simulink library "wtd_library_ver1"  (R2014b)
settings: Solver=ode45  StartTime=0.0  StopTime=10.0  RelTol=1e-3
undefined symbols (not defined in the file or in its folder): clearaugYMatrix, complexPower, dwo, faultaugYMatrix, genTranReactance, invclearaugYMatrix, invfaultaugYMatrix, invsystemaugYMatrix, j, nodeVoltage, noGridNodes, pffault_set_global, s3cc, tho
undefined symbols (not defined in the file): baseSystemPower, internalGenVoltage, pitchAngleVec, systemFrequency, turbSpeedVec, windturbKaParam, windturbKbParam, WTD_Y12, WTD_Y12_2
libraries: simulink x18
(part 2 of 3)

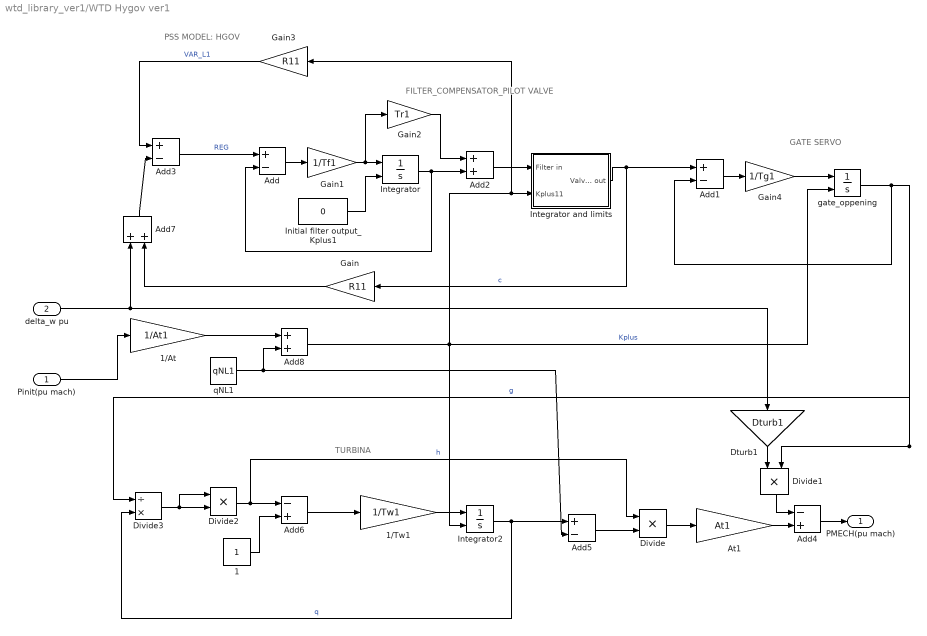
== system wtd_library_ver1/WTD Hygov ver1 ==
  note: GATE SERVO
  note: FILTER_COMPENSATOR_PILOT VALVE
  note: TURBINA
  note: PSS MODEL: HGOV
  Pinit(pu mach) : Inport
  delta_w pu : Inport  Port=2
  1 : Constant
  1/At : Gain  Gain=1/At1
  1/Tw1 : Gain  Gain=1/Tw1
  Add{,1,3,5} (4 alike) : Sum  Inputs=+-
  Add2 : Sum
  Add4 : Sum  Inputs=-+
  Add6 : Sum  Inputs=-+
  Add7 : Sum
  Add8 : Sum
  At1 : Gain  Gain=At1
  Divide : Product  Inputs=**
  Divide1 : Product  Inputs=**
  Divide2 : Product  Inputs=**
  Divide3 : Product  Inputs=/*
  Dturb1 : Gain  Gain=Dturb1
  Gain : Gain  Gain=R11
  Gain1 : Gain  Gain=1/Tf1
  Gain2 : Gain  Gain=Tr1
  Gain3 : Gain  Gain=R11
  Gain4 : Gain  Gain=1/Tg1
  Initial filter output_Kplus1 : Constant  Value=0
  Integrator : Integrator  InitialConditionSource=external  UpperSaturationLimit=VELM1  LowerSaturationLimit=-VELM1
  Integrator and limits : Subsystem
  Integrator2 : Integrator  InitialConditionSource=external
  gate_oppening : Integrator  InitialConditionSource=external
  qNL1 : Constant  Value=qNL1
  PMECH(pu mach) : Outport
  wires:
  Gain3/1 -> Add3/1  "VAR_L1"
  Add8/1 -> Gain3/1, Integrator and limits/2(Kplus11), gate_oppening/2, Integrator2/2  "Kplus"
  1/At/1 -> Add8/1
  Pinit(pu mach)/1 -> 1/At/1
  Gain2/1 -> Add2/1
  Add2/1 -> Integrator and limits/1(Filter in)
  Add/1 -> Gain1/1
  Gain1/1 -> Gain2/1, Integrator/1
  Initial filter output_Kplus1/1 -> Integrator/2
  Integrator/1 -> Add2/2, Add/2
  At1/1 -> Add4/2
  Add4/1 -> PMECH(pu mach)/1
  Divide/1 -> At1/1
  Divide1/1 -> Add4/1
  Add5/1 -> Divide/2
  1/Tw1/1 -> Integrator2/1
  qNL1/1 -> Add8/2, Add5/2
  Integrator2/1 -> Add5/1, Divide3/2  "q"
  Add6/1 -> 1/Tw1/1
  1/1 -> Add6/2
  Divide2/1 -> Add6/1, Divide/1  "h"
  Divide3/1 -> Divide2/2, Divide2/1
  Gain4/1 -> gate_oppening/1
  Add1/1 -> Gain4/1
  Integrator and limits/1(Valve out) -> Add1/1, Gain/1  "c"
  gate_oppening/1 -> Add1/2, Divide3/1, Divide1/2  "g"
  Add3/1 -> Add/1  "REG"
  Add7/1 -> Add3/2
  delta_w pu/1 -> Add7/1, Dturb1/1
  Gain/1 -> Add7/2
  Dturb1/1 -> Divide1/1

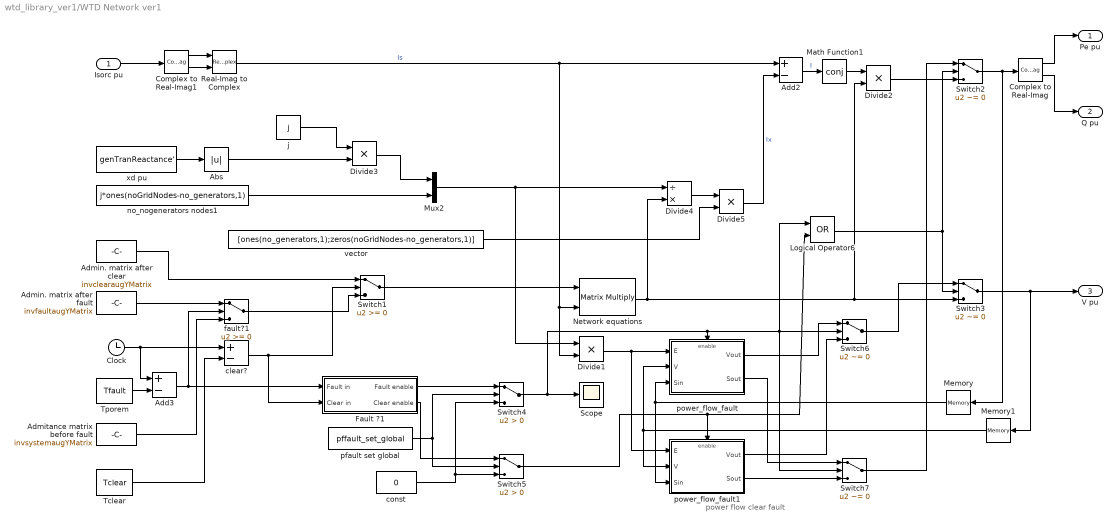
== system wtd_library_ver1/WTD Network ver1 ==
  note: power flow clear fault
  Isorc pu : Inport  OutDataTypeStr=double
  Abs : Abs
  Add2 : Sum  Inputs=+-
  Add3 : Sum  Inputs=+-
  Admin. matrix after fault : Constant  Value=invfaultaugYMatrix
  Admin. matrix after clear : Constant  Value=invclearaugYMatrix
  Admitance matrix before fault : Constant  Value=invsystemaugYMatrix
  Clock : Clock
  Complex to Real-Imag : ComplexToRealImag
  Complex to Real-Imag1 : ComplexToRealImag
  Divide{1..3,5} (4 alike) : Product  Inputs=**
  Divide4 : Product  Inputs=/*
  Fault ?1 : Subsystem
  Logical Operator6 : Logic  Operator=OR  AllPortsSameDT=off  OutDataTypeStr=boolean
  Math Function1 : Math  Operator=conj  SaturateOnIntegerOverflow=on
  Memory : Memory  X0=complexPower
  Memory1 : Memory  X0=nodeVoltage
  Mux2 : Mux  Inputs=2
  Network equations : Product  Inputs=**  Multiplication=Matrix(*)
  Real-Imag to Complex : RealImagToComplex
  Scope : Scope
      settings: MaxDataPoints=50000
  Switch1 : Switch
  Switch{2..3,6..7} (4 alike) : Switch  Criteria=u2 ~= 0
  Switch4 : Switch  Criteria=u2 > Threshold
  Switch5 : Switch  Criteria=u2 > Threshold
  Tclear : Constant  Value=Tclear
  Tporem : Constant  Value=Tfault
  clear? : Sum  Inputs=+-
  const : Constant  Value=0
  fault?1 : Switch
  j : Constant  Value=j
  no_nogenerators nodes1 : Constant  Value=j*ones(noGridNodes-no_generators,1)
  pfault set global : Constant  Value=pffault_set_global
  power_flow_fault : Subsystem
  power_flow_fault1 : Subsystem
  vector : Constant  Value=[ones(no_generators,1);zeros(noGridNodes-no_generators,1)]  VectorParams1D=off
  xd pu : Constant  Value=genTranReactance'
  Pe pu : Outport
  Q pu : Outport  Port=2
  V pu : Outport  Port=3
  wires:
  Divide1/1 -> power_flow_fault/1(E), power_flow_fault1/1(E)
  Divide3/1 -> Mux2/1
  no_nogenerators nodes1/1 -> Mux2/2
  Complex to Real-Imag/2 -> Q pu/1
  Complex to Real-Imag/1 -> Pe pu/1
  Math Function1/1 -> Divide2/1
  Add2/1 -> Math Function1/1  "I"
  Divide5/1 -> Add2/2  "Ix"
  vector/1 -> Divide5/2
  Divide4/1 -> Divide5/1
  Switch1/1 -> Network equations/1
  fault?1/1 -> Switch1/3
  clear?/1 -> Fault ?1/2(Clear in), Switch1/2
  Admin. matrix after clear/1 -> Switch1/1
  Tclear/1 -> clear?/2
  Add3/1 -> fault?1/2, Fault ?1/1(Fault in)
  Tporem/1 -> Add3/2
  Clock/1 -> Add3/1, clear?/1
  Admitance matrix before fault/1 -> fault?1/3
  Admin. matrix after fault/1 -> fault?1/1
  j/1 -> Divide3/1
  Abs/1 -> Divide3/2
  Mux2/1 -> Divide1/1, Divide4/1
  Network equations/1 -> Divide4/2, Divide2/2, Switch3/3
  xd pu/1 -> Abs/1
  Isorc pu/1 -> Complex to Real-Imag1/1
  Complex to Real-Imag1/1 -> Real-Imag to Complex/1
  Complex to Real-Imag1/2 -> Real-Imag to Complex/2
  Real-Imag to Complex/1 -> Add2/1, Network equations/2, Divide1/2  "Is"
  Divide2/1 -> Switch2/3
  Switch2/1 -> Complex to Real-Imag/1, Memory/1
  Switch3/1 -> V pu/1, Memory1/1
  const/1 -> Switch4/3, Switch5/3
  pfault set global/1 -> Switch4/2, Switch5/2
  Switch4/1 -> power_flow_fault/Enable, Logical Operator6/1, Switch6/2, Switch7/2, Scope/1
  Memory/1 -> power_flow_fault/3(Sin), power_flow_fault1/3(Sin)
  Memory1/1 -> power_flow_fault/2(V), power_flow_fault1/2(V)
  Switch5/1 -> power_flow_fault1/Enable, Logical Operator6/2
  Logical Operator6/1 -> Switch2/2, Switch3/2
  power_flow_fault/1(Vout) -> Switch6/1
  power_flow_fault1/1(Vout) -> Switch6/3
  power_flow_fault/2(Sout) -> Switch7/1
  power_flow_fault1/2(Sout) -> Switch7/3
  Switch6/1 -> Switch3/1
  Switch7/1 -> Switch2/1
  Fault ?1/1(Fault enable) -> Switch4/1
  Fault ?1/2(Clear enable) -> Switch5/1

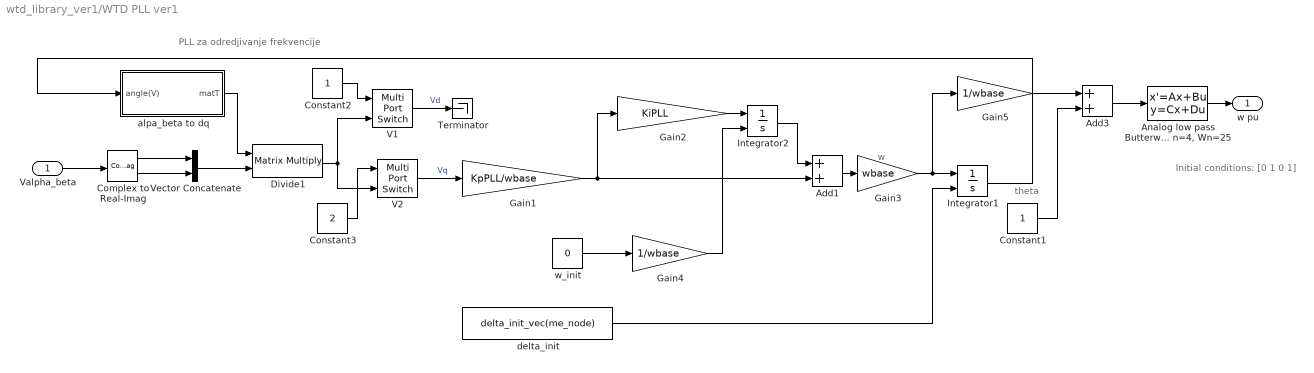
== system wtd_library_ver1/WTD PLL ver1 ==
  note: PLL za odredjivanje frekvencije
  note: theta
  note: w
  note: Initial conditions:
      | [0 1 0 1]
  Valpha_beta : Inport
  Add1 : Sum
  Add3 : Sum
  "Analog low pass Butterworth filter, n=4, Wn=25" : StateSpace  A=[-46.194,-25,0,0;25,0,0,0;0,25,-19.134,-25;0,0,25,0]  B=[25;0;0;0]  C=[0,0,0,1]  D=0  X0=[0 1 0 1]
  Complex to Real-Imag : ComplexToRealImag
  Constant1 : Constant
  Constant2 : Constant
  Constant3 : Constant  Value=2
  Divide1 : Product  Inputs=**  Multiplication=Matrix(*)
  Gain1 : Gain  Gain=KpPLL/wbase
  Gain2 : Gain  Gain=KiPLL
  Gain3 : Gain  Gain=wbase
  Gain4 : Gain  Gain=1/wbase
  Gain5 : Gain  Gain=1/wbase
  Integrator1 : Integrator  InitialConditionSource=external
  Integrator2 : Integrator  InitialConditionSource=external
  Terminator : Terminator
  V1 : MultiPortSwitch  Inputs=1
  V2 : MultiPortSwitch  Inputs=1
  Vector Concatenate : Concatenate
  alpa_beta to dq : Subsystem
  delta_init : Constant  Value=delta_init_vec(me_node)
  w_init : Constant  Value=0
  w pu : Outport
  wires:
  "Analog low pass Butterworth filter, n=4, Wn=25"/1 -> w pu/1
  Add3/1 -> "Analog low pass Butterworth filter, n=4, Wn=25"/1
  Valpha_beta/1 -> Complex to Real-Imag/1
  alpa_beta to dq/1(matT) -> Divide1/1
  Vector Concatenate/1 -> Divide1/2
  Complex to Real-Imag/1 -> Vector Concatenate/1
  Complex to Real-Imag/2 -> Vector Concatenate/2
  Gain1/1 -> Gain2/1, Add1/2
  Integrator1/1 -> alpa_beta to dq/1(angle(V))
  Constant2/1 -> V1/1
  Constant3/1 -> V2/1
  V1/1 -> Terminator/1  "Vd"
  Add1/1 -> Gain3/1
  Integrator2/1 -> Add1/1
  Gain2/1 -> Integrator2/1
  V2/1 -> Gain1/1  "Vq"
  Gain3/1 -> Integrator1/1, Gain5/1
  delta_init/1 -> Integrator1/2
  Gain4/1 -> Integrator2/2
  Gain5/1 -> Add3/1
  Constant1/1 -> Add3/2
  Divide1/1 -> V1/2, V2/2
  w_init/1 -> Gain4/1

== system wtd_library_ver1/WTD Rotor ver1 ==
  note: This subsystem models the mechanical part of the synchronous machine (Kundur)
  "deltaPe pu mach " : Inport  PortDimensions=1
  deltaPm pu mach : Inport  Port=2  PortDimensions=1
  initial_angle(elrad) : Inport  Port=3  PortDimensions=1
  delta_w_init pu : Inport  Port=4  PortDimensions=1
  Constant : Constant
  F1 : Gain  Gain=D  SaturateOnIntegerOverflow=on  OutDataTypeStr=Inherit: Same as input  ParamDataTypeStr=Inherit: Same as input
  H : Constant  Value=H
  Integrator : Integrator  InitialConditionSource=external  InitialCondition=dwo
  Integrator2 : Integrator  InitialConditionSource=external  InitialCondition=tho
  Product1 : Product  Inputs=*/  SaturateOnIntegerOverflow=on  InputSameDT=on  OutDataTypeStr=Inherit: Same as first input
  Product2 : Product  Inputs=*/  SaturateOnIntegerOverflow=on  InputSameDT=on  OutDataTypeStr=Inherit: Same as first input
  Sum1 : Sum  Inputs=+-  SaturateOnIntegerOverflow=on  InputSameDT=on  OutDataTypeStr=Inherit: Same as first input
  Sum2 : Sum  Inputs=+-  SaturateOnIntegerOverflow=on  InputSameDT=on  OutDataTypeStr=Inherit: Same as first input
  Sum3 : Sum  SaturateOnIntegerOverflow=on  InputSameDT=on  OutDataTypeStr=Inherit: Same as first input
  gain : Gain  Gain=2  SaturateOnIntegerOverflow=on  OutDataTypeStr=Inherit: Same as input  ParamDataTypeStr=Inherit: Same as input
  wbase : Gain  Gain=wbase  SaturateOnIntegerOverflow=on  OutDataTypeStr=Inherit: Same as input  ParamDataTypeStr=Inherit: Same as input
  angle(elrad) : Outport  InitialOutput=0
  "delta_w pu " : Outport  Port=2  InitialOutput=0
  wires:
  "deltaPe pu mach "/1 -> Sum2/2  "Pe"
  Product1/1 -> Integrator/1
  Integrator/1 -> wbase/1, F1/1, "delta_w pu "/1, Sum3/2  "dw"
  wbase/1 -> Integrator2/1  "delta_w"
  Integrator2/1 -> angle(elrad)/1  "delta (rad)"
  initial_angle(elrad)/1 -> Integrator2/2
  delta_w_init pu/1 -> Integrator/2
  H/1 -> gain/1
  gain/1 -> Product1/2
  Sum1/1 -> Product1/1
  F1/1 -> Sum1/2
  Sum2/1 -> Product2/1
  Product2/1 -> Sum1/1
  Constant/1 -> Sum3/1
  Sum3/1 -> Product2/2
  deltaPm pu mach/1 -> Sum2/1

== system wtd_library_ver1/WTD Tgov1 ver1 ==
  note: MODEL PSS: TGOV1
  Pinit(pu mach) : Inport
  delta_w pu : Inport  Port=2
  Add : Sum  Inputs=+-
  Add1 : Sum  Inputs=+-
  Add2 : Sum  Inputs=++-
  Add3 : Sum  Inputs=+-
  Gain : Gain  Gain=1/R2
  Gain1 : Gain  Gain=1/T12
  Gain2 : Gain  Gain=1/T32
  Gain3 : Gain  Gain=T22
  Gain4 : Gain  Gain=Dt2
  Gain5 : Gain  Gain=R2
  Integrator : Integrator  InitialConditionSource=external  LimitOutput=on  UpperSaturationLimit=Vmax2  LowerSaturationLimit=Vmin2
  Integrator1 : Integrator  InitialConditionSource=external
  PMECH(pu mach) : Outport
  wires:
  Pinit(pu mach)/1 -> Gain5/1, Integrator/2, Integrator1/2
  Gain5/1 -> Add3/1
  Add3/1 -> Gain/1
  delta_w pu/1 -> Add3/2, Gain4/1
  Gain4/1 -> Add2/3
  Add2/1 -> PMECH(pu mach)/1
  Gain3/1 -> Add2/1
  Integrator1/1 -> Add2/2, Add1/2
  Gain2/1 -> Gain3/1, Integrator1/1
  Add1/1 -> Gain2/1
  Integrator/1 -> Add1/1, Add/2
  Gain1/1 -> Integrator/1
  Add/1 -> Gain1/1
  Gain/1 -> Add/1

== system wtd_library_ver1/WTD Thermo ver1 ==
  note: STEAM 2
  Pe pu : Inport
  Add4 : Sum  Inputs=+-
  Add5 : Sum  Inputs=+-
  Gain1 : Gain  Gain=1/Sbasem2
  Gain2 : Gain  Gain=Sbasesys/Sbasem2
  Gain3 : Gain  Gain=Sbasem2/Sbasesys
  Pm_init : Constant  Value=Pm_init_vec(co_node)
  Rotor/Load1 : Subsystem
  TGOV1 : Subsystem
  delta_init (elrad) : Constant  Value=delta_init_vec(co_node)
  delta_w2 : Constant  Value=0
  Pm pu : Outport
  angle(elrad) : Outport  Port=2
  delta_w pu : Outport  Port=3
  wires:
  Pm_init/1 -> Gain1/1
  TGOV1/1(PMECH) -> Gain3/1, Add4/1
  Add5/1 -> Rotor/Load1/1("deltaPe(pu) ")
  Add4/1 -> Rotor/Load1/2(deltaPm(pu))
  Rotor/Load1/2(delta_w(pu)) -> TGOV1/2(deltaw), delta_w pu/1
  delta_w2/1 -> Rotor/Load1/4(deltawro)
  Gain2/1 -> Add5/1
  Pe pu/1 -> Gain2/1
  Gain3/1 -> Pm pu/1
  Rotor/Load1/1(delta(elrad)) -> angle(elrad)/1
  delta_init (elrad)/1 -> Rotor/Load1/3(angle(E)(elrad))
  Gain1/1 -> Add4/2, Add5/2, TGOV1/1(Pinit (pu mach))

== system wtd_library_ver1/WTD Vec_ sig_sel ver1 ==
  in : Inport
  V7 : MultiPortSwitch  Inputs=1
  signal node : Constant  Value=node
  out : Outport
  wires:
  in/1 -> V7/2
  V7/1 -> out/1
  signal node/1 -> V7/1

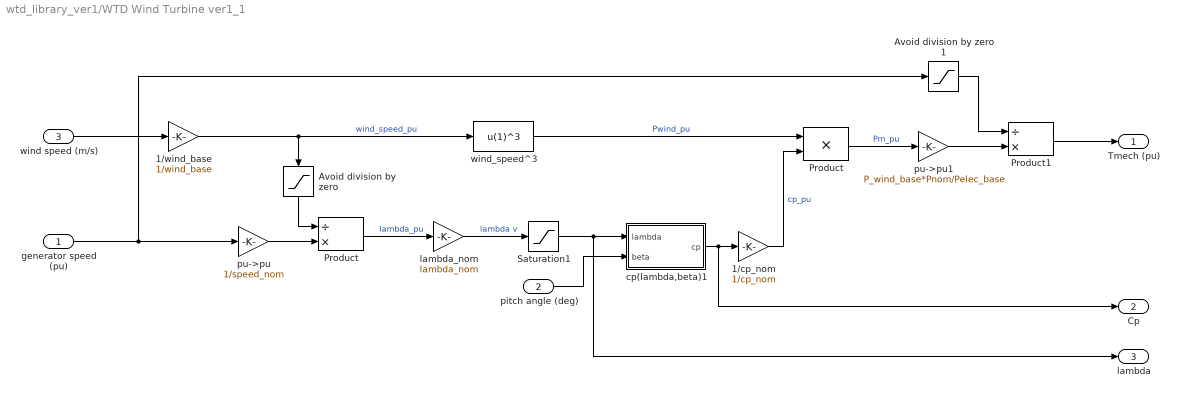
== system wtd_library_ver1/WTD Wind Turbine ver1_1 ==
  generator speed (pu) : Inport
  pitch angle (deg) : Inport  Port=2
  wind speed (m/s) : Inport  Port=3
  1/cp_nom : Gain  Gain=1/cp_nom  SaturateOnIntegerOverflow=on  OutDataTypeStr=Inherit: Same as input  ParamDataTypeStr=Inherit: Same as input
  1/wind_base : Gain  Gain=1/wind_base  SaturateOnIntegerOverflow=on  OutDataTypeStr=Inherit: Same as input  ParamDataTypeStr=Inherit: Same as input
  "Avoid division by zero " : Saturate  UpperLimit=1e6  LowerLimit=1e-6
  Avoid division by zero 1 : Saturate  UpperLimit=1e6  LowerLimit=1e-6
  Product : Product  Inputs=/*  SaturateOnIntegerOverflow=on  OutDataTypeStr=Inherit: Same as first input
  "Product " : Product  SaturateOnIntegerOverflow=on  OutDataTypeStr=Inherit: Same as first input
  Product1 : Product  Inputs=/*  SaturateOnIntegerOverflow=on  OutDataTypeStr=Inherit: Same as first input
  Saturation1 : Saturate  UpperLimit=inf  LowerLimit=1e-6
  cp(lambda,beta)1 : Subsystem
  lambda_nom : Gain  Gain=lambda_nom  SaturateOnIntegerOverflow=on  OutDataTypeStr=Inherit: Same as input  ParamDataTypeStr=Inherit: Same as input
  "pu->pu " : Gain  Gain=1/speed_nom  SaturateOnIntegerOverflow=on  OutDataTypeStr=Inherit: Same as input  ParamDataTypeStr=Inherit: Same as input
  pu->pu1 : Gain  Gain=P_wind_base*Pnom/Pelec_base  SaturateOnIntegerOverflow=on  OutDataTypeStr=Inherit: Same as input  ParamDataTypeStr=Inherit: Same as input
  wind_speed^3 : Fcn  Expr=u(1)^3
  Tmech (pu) : Outport
  Cp : Outport  Port=2
  lambda : Outport  Port=3
  wires:
  wind speed (m/s)/1 -> 1/wind_base/1
  "pu->pu "/1 -> Product/2
  "Avoid division by zero "/1 -> Product/1
  1/wind_base/1 -> "Avoid division by zero "/1, wind_speed^3/1  "wind_speed_pu"
  Product/1 -> lambda_nom/1  "lambda_pu"
  Saturation1/1 -> cp(lambda,beta)1/1(lambda), lambda/1
  1/cp_nom/1 -> "Product "/2  "cp_pu"
  lambda_nom/1 -> Saturation1/1  "lambda v"
  generator speed (pu)/1 -> "pu->pu "/1, Avoid division by zero 1/1
  wind_speed^3/1 -> "Product "/1  "Pwind_pu"
  cp(lambda,beta)1/1(cp) -> Cp/1, 1/cp_nom/1
  pitch angle (deg)/1 -> cp(lambda,beta)1/2(beta)
  Avoid division by zero 1/1 -> Product1/1
  Product1/1 -> Tmech (pu)/1
  pu->pu1/1 -> Product1/2
  "Product "/1 -> pu->pu1/1  "Pm_pu"

== system wtd_library_ver1/WTD zero_gen ver1 ==
  Complex to Real-Imag : ComplexToRealImag
  Constant : Constant  Value=0
  Real-Imag to Complex : RealImagToComplex
  Isorc : Outport
  wires:
  Real-Imag to Complex/1 -> Isorc/1
  Complex to Real-Imag/2 -> Real-Imag to Complex/2
  Complex to Real-Imag/1 -> Real-Imag to Complex/1
  Constant/1 -> Complex to Real-Imag/1

== system wtd_library_ver1/WTD DFIG_ver1/Calculation of Power to network  ==
  absVterm : Inport
  Vterm : Inport  Port=2
  Isorc : Inport  Port=3
  Xsec : Inport  Port=4
  Add1 : Sum  Inputs=+-
  Complex to Real-Imag1 : ComplexToRealImag  Output=Real
  Complex to Real-Imag2 : ComplexToRealImag  Output=Imag
  Divide : Product  Inputs=**
  Divide1 : Product  Inputs=*/
  Divide4 : Product  Inputs=**
  Gain1 : Gain  Gain=-1
  Math Function : Math  Operator=conj  SaturateOnIntegerOverflow=on
  Math Function1 : Math  Operator=square  SaturateOnIntegerOverflow=on
  j : Constant  Value=j
  Pgen=Pelec : Outport
  Qgen : Outport  Port=2
  Sgen : Outport  Port=3
  wires:
  Gain1/1 -> Divide1/2
  Divide4/1 -> Gain1/1
  j/1 -> Divide4/2
  Math Function1/1 -> Divide1/1
  Divide1/1 -> Add1/2
  Divide/1 -> Complex to Real-Imag1/1, Add1/1  "Selec"
  Add1/1 -> Complex to Real-Imag2/1, Sgen/1  "Sgen (after Xsec)"
  Math Function/1 -> Divide/2
  absVterm/1 -> Math Function1/1
  Vterm/1 -> Divide/1
  Isorc/1 -> Math Function/1
  Xsec/1 -> Divide4/1
  Complex to Real-Imag1/1 -> Pgen=Pelec/1  "Pelec"
  Complex to Real-Imag2/1 -> Qgen/1

== system wtd_library_ver1/WTD DFIG_ver1/Converter control model ==
  note: Measurements
  Vrfq : Inport
  Vreg : Inport  Port=2
  Qord_sep_mod : Inport  Port=3
  PFAref : Inport  Port=4
  Pelec : Inport  Port=5
  Qgen : Inport  Port=6
  Vterm : Inport  Port=7
  Pord : Inport  Port=8
  Qinput_droop : Inport  Port=9
  Qref : Inport  Port=10
  Aux_Test_Sig : Inport  Port=11
  Electrical Control : Subsystem
  Reactive Power Control : Subsystem
  Eqcmd : Outport
  Ipcmd : Outport  Port=2
  wires:
  Electrical Control/2(Ipcmd) -> Ipcmd/1
  Electrical Control/1(Eqcmd) -> Eqcmd/1
  Aux_Test_Sig/1 -> Electrical Control/5(Aux_Test_Sig)
  Pord/1 -> Electrical Control/4(Pord)
  Vterm/1 -> Electrical Control/3(Vterm)
  Qgen/1 -> Electrical Control/2(Qgen)
  Reactive Power Control/1(Qcmd) -> Electrical Control/1(Qcmd)
  Qinput_droop/1 -> Reactive Power Control/6(Qinput_droop)
  Qref/1 -> Reactive Power Control/7(Qref)
  Pelec/1 -> Reactive Power Control/5(Pelec)
  PFAref/1 -> Reactive Power Control/4(PFAref)
  Qord_sep_mod/1 -> Reactive Power Control/3(Qord_sep_mod)
  Vreg/1 -> Reactive Power Control/2(Vreg)
  Vrfq/1 -> Reactive Power Control/1(Vrfq)

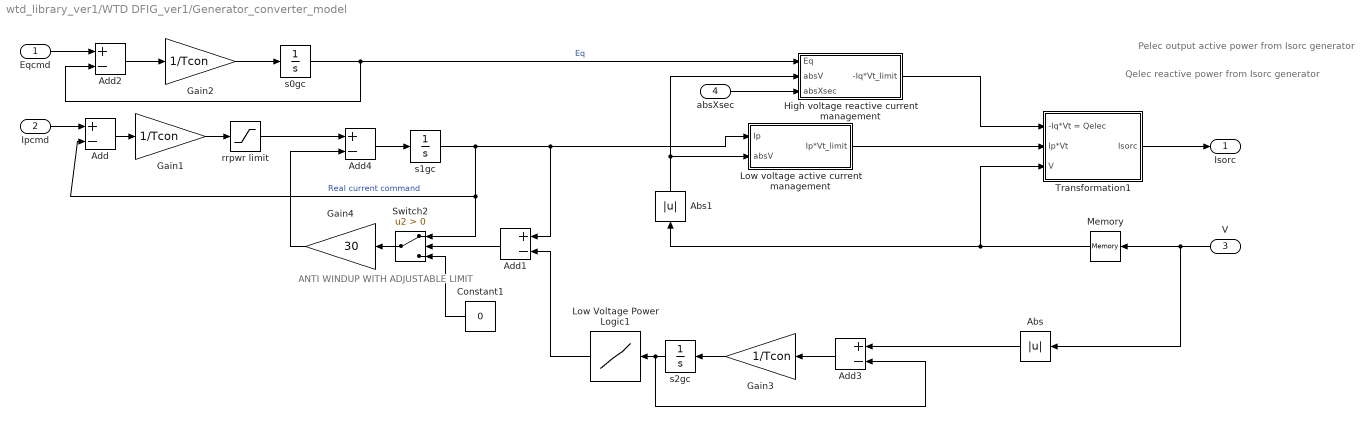
== system wtd_library_ver1/WTD DFIG_ver1/Generator_converter_model ==
  note: Pelec output active power from Isorc generator
  note: Qelec reactive power from Isorc generator
  note: ANTI WINDUP WITH ADJUSTABLE
      | LIMIT
  Eqcmd : Inport
  Ipcmd : Inport  Port=2
  V : Inport  Port=3
  absXsec : Inport  Port=4
  " Transformation1" : Subsystem
  Abs : Abs
  Abs1 : Abs
  Add{,1..4} (5 alike) : Sum  Inputs=+-
  Constant1 : Constant  Value=0
  Gain1 : Gain  Gain=1/Tcon
  Gain2 : Gain  Gain=1/Tcon
  Gain3 : Gain  Gain=1/Tcon
  Gain4 : Gain  Gain=30
  High voltage reactive current management : Subsystem
  Low Voltage Power Logic1 : Lookup  InputValues=[0,zerox,brkpt,brkpt+eps,brkpt+2*eps]  Table=[0 0 1.22 2 2]
  Low voltage active current management : Subsystem
  Memory : Memory  X0=nodeVoltage(co_node)
  Switch2 : Switch  Criteria=u2 > Threshold
  rrpwr limit : Saturate  UpperLimit=rrpwr  LowerLimit=-inf
  s0gc : Integrator  InitialCondition=s0gc
  s1gc : Integrator  InitialCondition=s1gc
  s2gc : Integrator  InitialCondition=s2gc
  Isorc : Outport
  wires:
  Abs/1 -> Add3/1
  " Transformation1"/1(Isorc) -> Isorc/1
  absXsec/1 -> High voltage reactive current management/3(absXsec)
  V/1 -> Abs/1, Memory/1
  Add3/1 -> Gain3/1
  s2gc/1 -> Add3/2, Low Voltage Power Logic1/1
  Gain3/1 -> s2gc/1
  s0gc/1 -> Add2/2, High voltage reactive current management/1(Eq)  "Eq"
  Gain2/1 -> s0gc/1
  Add2/1 -> Gain2/1
  Eqcmd/1 -> Add2/1
  Ipcmd/1 -> Add/1
  Add/1 -> Gain1/1
  Gain1/1 -> rrpwr limit/1
  High voltage reactive current management/1(-Iq*Vt_limit) -> " Transformation1"/1(-Iq*Vt = Qelec)
  Low voltage active current management/1(Ip*Vt_limit) -> " Transformation1"/2(Ip*Vt)
  Abs1/1 -> Low voltage active current management/2(absV), High voltage reactive current management/2(absV)
  s1gc/1 -> Add/2, Switch2/1, Low voltage active current management/1(Ip), Add1/1  "Real current command"
  Memory/1 -> " Transformation1"/3(V), Abs1/1
  rrpwr limit/1 -> Add4/1
  Add4/1 -> s1gc/1
  Switch2/1 -> Gain4/1
  Constant1/1 -> Switch2/3
  Gain4/1 -> Add4/2
  Low Voltage Power Logic1/1 -> Add1/2
  Add1/1 -> Switch2/2

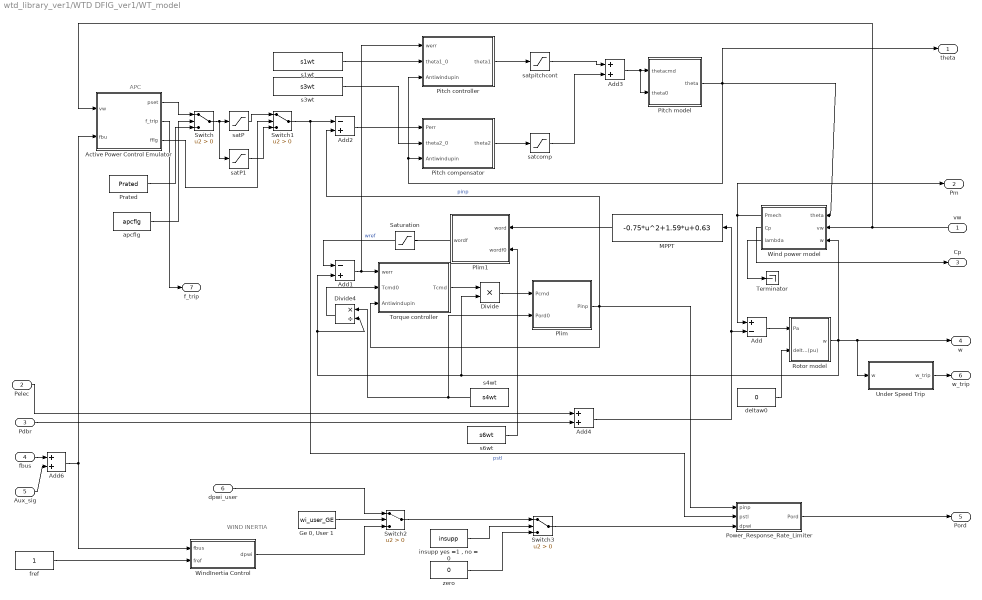
== system wtd_library_ver1/WTD DFIG_ver1/WT_model ==
  note: WIND INERTIA
  note: APC
  vw : Inport
  Pelec : Inport  Port=2
  Pdbr : Inport  Port=3
  fbus : Inport  Port=4
  Aux_sig : Inport  Port=5
  dpwi_user : Inport  Port=6
  Active Power Control Emulator : Subsystem
  Add : Sum  Inputs=+-
  Add1 : Sum  Inputs=-+
  Add2 : Sum  Inputs=-+
  Add3 : Sum
  Add4 : Sum
  Add6 : Sum
  Divide : Product  Inputs=**
  Divide4 : Product  Inputs=*/
  "Ge 0, User 1" : Constant  Value=wi_user_GE
  MPPT : Fcn  Expr=-0.75*u^2+1.59*u+0.63
  Pitch compensator : Subsystem
  Pitch controller : Subsystem
  Pitch model : Subsystem
  Plim : Subsystem
  Plim1 : Subsystem
  Power_Response_Rate_Limiter : Subsystem
  Prated : Constant  Value=Prated
  Rotor model : Subsystem
  Saturation : Saturate  UpperLimit=wrefgr  LowerLimit=0.63
  Switch{,1..3} (4 alike) : Switch  Criteria=u2 > Threshold
  Terminator : Terminator
  Torque controller : Subsystem
  Under Speed Trip : Subsystem
  Wind power model : Subsystem
  WindInertia Control : Subsystem
  apcflg : Constant  Value=apcflg
  deltaw0 : Constant  Value=0
  fref : Constant
  "insupp yes =1 , no = 0" : Constant  Value=insupp
  s1wt : Constant  Value=s1wt
  s3wt : Constant  Value=s3wt
  s4wt : Constant  Value=s4wt
  s6wt : Constant  Value=s6wt
  satP : Saturate  UpperLimit=+inf  LowerLimit=Pmin
  satP1 : Saturate  UpperLimit=Pmax  LowerLimit=Pmin
  satcomp : Saturate  UpperLimit=upltpitchcomp  LowerLimit=lowltpitchcomp
  satpitchcont : Saturate  UpperLimit=upltpitchcont  LowerLimit=lowltpitchcont
  zero : Constant  Value=0
  theta : Outport
  Pm : Outport  Port=2
  Cp : Outport  Port=3
  w : Outport  Port=4
  Pord : Outport  Port=5
  w_trip : Outport  Port=6
  f_trip : Outport  Port=7
  wires:
  Switch3/1 -> Power_Response_Rate_Limiter/3(dpwi)
  zero/1 -> Switch3/3
  Switch2/1 -> Switch3/1
  "insupp yes =1 , no = 0"/1 -> Switch3/2
  deltaw0/1 -> Rotor model/2(deltaw0(pu))
  Power_Response_Rate_Limiter/1(Pord) -> Pord/1
  fref/1 -> WindInertia Control/2(fref)
  WindInertia Control/1(dpwi) -> Switch2/3
  dpwi_user/1 -> Switch2/1
  satP1/1 -> Switch1/3
  satP/1 -> Switch1/1
  Switch1/1 -> Power_Response_Rate_Limiter/2(pstl), Add2/1  "pstl"
  Active Power Control Emulator/3(fflg) -> Switch1/2
  Active Power Control Emulator/2(f_trip) -> f_trip/1
  Under Speed Trip/1(w_trip) -> w_trip/1
  Aux_sig/1 -> Add6/2
  Pdbr/1 -> Add4/2
  Pelec/1 -> Add4/1
  Wind power model/2(Cp) -> Cp/1
  apcflg/1 -> Switch/2
  Prated/1 -> Switch/3
  Active Power Control Emulator/1(pset) -> Switch/1
  Switch/1 -> satP1/1, satP/1
  Add6/1 -> WindInertia Control/1(fbus), Active Power Control Emulator/2(fbu)
  fbus/1 -> Add6/1
  Wind power model/3(lambda) -> Terminator/1
  Add4/1 -> Add/2, MPPT/1
  satcomp/1 -> Add3/2
  satpitchcont/1 -> Add3/1
  Plim1/1(wordf) -> Saturation/1
  MPPT/1 -> Plim1/1(word)
  vw/1 -> Wind power model/2(vw), Active Power Control Emulator/1(vw)
  s1wt/1 -> Pitch controller/2(theta1_0)
  s3wt/1 -> Pitch compensator/2(theta2_0)
  Divide4/1 -> Torque controller/2(Tcmd0)
  s6wt/1 -> Plim1/2(wordf0)
  s4wt/1 -> Plim/2(Pord0), Divide4/1
  Plim/1(Pinp) -> Power_Response_Rate_Limiter/1(pinp), Torque controller/3(Antiwindupin), Add2/2  "pinp"
  Wind power model/1(Pmech) -> Add/1, Pm/1
  Pitch model/1(theta) -> theta/1, Pitch compensator/3(Antiwindupin), Pitch controller/3(Antiwindupin), Wind power model/1(theta)
  Add3/1 -> Pitch model/2(theta0), Pitch model/1(thetacmd)
  Pitch compensator/1(theta2) -> satcomp/1
  Pitch controller/1(theta1) -> satpitchcont/1
  Add2/1 -> Pitch compensator/1(Perr)
  Saturation/1 -> Add1/1  "wref"
  Add1/1 -> Pitch controller/1(werr), Torque controller/1(werr)
  Torque controller/1(Tcmd) -> Divide/1
  Rotor model/1(w) -> Under Speed Trip/1(w), w/1, Divide4/2, Add1/2, Divide/2, Wind power model/3(w)
  Divide/1 -> Plim/1(Pcmd)
  Add/1 -> Rotor model/1(Pa)
  "Ge 0, User 1"/1 -> Switch2/2

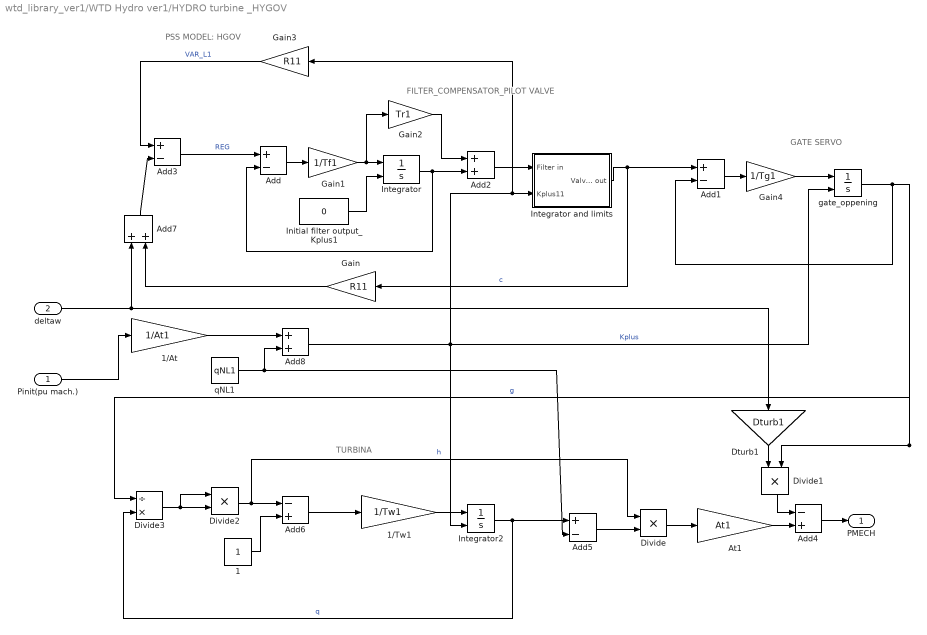
== system wtd_library_ver1/WTD Hydro ver1/HYDRO turbine _HYGOV ==
  note: GATE SERVO
  note: FILTER_COMPENSATOR_PILOT VALVE
  note: TURBINA
  note: PSS MODEL: HGOV
  Pinit(pu mach.) : Inport
  deltaw : Inport  Port=2
  1 : Constant
  1/At : Gain  Gain=1/At1
  1/Tw1 : Gain  Gain=1/Tw1
  Add{,1,3,5} (4 alike) : Sum  Inputs=+-
  Add2 : Sum
  Add4 : Sum  Inputs=-+
  Add6 : Sum  Inputs=-+
  Add7 : Sum
  Add8 : Sum
  At1 : Gain  Gain=At1
  Divide : Product  Inputs=**
  Divide1 : Product  Inputs=**
  Divide2 : Product  Inputs=**
  Divide3 : Product  Inputs=/*
  Dturb1 : Gain  Gain=Dturb1
  Gain : Gain  Gain=R11
  Gain1 : Gain  Gain=1/Tf1
  Gain2 : Gain  Gain=Tr1
  Gain3 : Gain  Gain=R11
  Gain4 : Gain  Gain=1/Tg1
  Initial filter output_Kplus1 : Constant  Value=0
  Integrator : Integrator  InitialConditionSource=external  UpperSaturationLimit=VELM1  LowerSaturationLimit=-VELM1
  Integrator and limits : Subsystem
  Integrator2 : Integrator  InitialConditionSource=external
  gate_oppening : Integrator  InitialConditionSource=external
  qNL1 : Constant  Value=qNL1
  PMECH : Outport
  wires:
  Gain3/1 -> Add3/1  "VAR_L1"
  Add8/1 -> Gain3/1, Integrator and limits/2(Kplus11), gate_oppening/2, Integrator2/2  "Kplus"
  1/At/1 -> Add8/1
  Pinit(pu mach.)/1 -> 1/At/1
  Gain2/1 -> Add2/1
  Add2/1 -> Integrator and limits/1(Filter in)
  Add/1 -> Gain1/1
  Gain1/1 -> Gain2/1, Integrator/1
  Initial filter output_Kplus1/1 -> Integrator/2
  Integrator/1 -> Add2/2, Add/2
  At1/1 -> Add4/2
  Add4/1 -> PMECH/1
  Divide/1 -> At1/1
  Divide1/1 -> Add4/1
  Add5/1 -> Divide/2
  1/Tw1/1 -> Integrator2/1
  qNL1/1 -> Add8/2, Add5/2
  Integrator2/1 -> Add5/1, Divide3/2  "q"
  Add6/1 -> 1/Tw1/1
  1/1 -> Add6/2
  Divide2/1 -> Add6/1, Divide/1  "h"
  Divide3/1 -> Divide2/2, Divide2/1
  Gain4/1 -> gate_oppening/1
  Add1/1 -> Gain4/1
  Integrator and limits/1(Valve out) -> Add1/1, Gain/1  "c"
  gate_oppening/1 -> Add1/2, Divide3/1, Divide1/2  "g"
  Add3/1 -> Add/1  "REG"
  Add7/1 -> Add3/2
  deltaw/1 -> Add7/1, Dturb1/1
  Gain/1 -> Add7/2
  Dturb1/1 -> Divide1/1

== system wtd_library_ver1/WTD Hydro ver1/Rotor//Load2 ==
  note: This subsystem models the mechanical part of the synchronous machine (Kundur)
  "deltaPe(pu) " : Inport  PortDimensions=1
  deltaPm(pu) : Inport  Port=2  PortDimensions=1
  angle(E)(elrad) : Inport  Port=3  PortDimensions=1
  deltawro : Inport  Port=4  PortDimensions=1
  Constant : Constant
  F1 : Gain  Gain=D1  SaturateOnIntegerOverflow=on  OutDataTypeStr=Inherit: Same as input  ParamDataTypeStr=Inherit: Same as input
  H : Constant  Value=H1
  Integrator : Integrator  InitialConditionSource=external  InitialCondition=dwo
  Integrator2 : Integrator  InitialConditionSource=external  InitialCondition=tho
  Product1 : Product  Inputs=*/  SaturateOnIntegerOverflow=on  InputSameDT=on  OutDataTypeStr=Inherit: Same as first input
  Product2 : Product  Inputs=*/  SaturateOnIntegerOverflow=on  InputSameDT=on  OutDataTypeStr=Inherit: Same as first input
  Sum1 : Sum  Inputs=+-  SaturateOnIntegerOverflow=on  InputSameDT=on  OutDataTypeStr=Inherit: Same as first input
  Sum2 : Sum  Inputs=+-  SaturateOnIntegerOverflow=on  InputSameDT=on  OutDataTypeStr=Inherit: Same as first input
  Sum3 : Sum  SaturateOnIntegerOverflow=on  InputSameDT=on  OutDataTypeStr=Inherit: Same as first input
  gain : Gain  Gain=2  SaturateOnIntegerOverflow=on  OutDataTypeStr=Inherit: Same as input  ParamDataTypeStr=Inherit: Same as input
  wbase : Gain  Gain=wbase  SaturateOnIntegerOverflow=on  OutDataTypeStr=Inherit: Same as input  ParamDataTypeStr=Inherit: Same as input
  delta(elrad) : Outport  InitialOutput=0
  delta_w(pu) : Outport  Port=2  InitialOutput=0
  wires:
  H/1 -> gain/1
  deltaPm(pu)/1 -> Sum2/1
  Sum3/1 -> Product2/2
  Constant/1 -> Sum3/1
  Product2/1 -> Sum1/1
  Sum2/1 -> Product2/1
  F1/1 -> Sum1/2
  Sum1/1 -> Product1/1
  gain/1 -> Product1/2
  deltawro/1 -> Integrator/2
  angle(E)(elrad)/1 -> Integrator2/2
  Integrator2/1 -> delta(elrad)/1  "delta (rad)"
  wbase/1 -> Integrator2/1  "delta_w"
  Integrator/1 -> Sum3/2, delta_w(pu)/1, F1/1, wbase/1  "dw"
  Product1/1 -> Integrator/1
  "deltaPe(pu) "/1 -> Sum2/2  "Pe"

== system wtd_library_ver1/WTD Hygov ver1/Integrator and limits ==
  Filter in : Inport
  Kplus11 : Inport  Port=2
  Gain2 : Gain  Gain=1/(r1*Tr1)
  Saturation : Saturate  UpperLimit=VELM1  LowerLimit=-VELM1
  gate_ref : Integrator  InitialConditionSource=external  LimitOutput=on  UpperSaturationLimit=Gmax1  LowerSaturationLimit=Gmin1
  Valve out : Outport
  wires:
  Filter in/1 -> Gain2/1
  Gain2/1 -> Saturation/1
  gate_ref/1 -> Valve out/1
  Saturation/1 -> gate_ref/1
  Kplus11/1 -> gate_ref/2

== system wtd_library_ver1/WTD Network ver1/Fault ?1 ==
  Fault in : Inport
  Clear in : Inport  Port=2
  Logical Operator1 : Logic  Operator=NOT  AllPortsSameDT=off  OutDataTypeStr=boolean
  Logical Operator2 : Logic  AllPortsSameDT=off  OutDataTypeStr=boolean
  Logical Operator5 : Logic  Operator=NOT  AllPortsSameDT=off  OutDataTypeStr=boolean
  Logical Operator6 : Logic  AllPortsSameDT=off  OutDataTypeStr=boolean
  Memory{,1..3} (4 alike) : Memory
  fault? : Switch
  fault?1 : Switch
  one const : Constant
  one const1 : Constant
  zero const : Constant  Value=0
  zero const1 : Constant  Value=0
  Fault enable : Outport
  Clear enable : Outport  Port=2
  wires:
  Fault in/1 -> fault?/2
  Memory/1 -> Memory2/1
  fault?/1 -> Memory/1, Logical Operator6/1
  zero const/1 -> fault?/3
  one const/1 -> fault?/1
  Clear in/1 -> fault?1/2
  one const1/1 -> fault?1/1
  zero const1/1 -> fault?1/3
  Memory2/1 -> Logical Operator5/1
  Logical Operator5/1 -> Logical Operator6/2
  Memory1/1 -> Memory3/1
  fault?1/1 -> Logical Operator2/1, Memory1/1
  Memory3/1 -> Logical Operator1/1
  Logical Operator1/1 -> Logical Operator2/2
  Logical Operator6/1 -> Fault enable/1
  Logical Operator2/1 -> Clear enable/1

== system wtd_library_ver1/WTD Network ver1/power_flow_fault ==
  E : Inport
  V : Inport  Port=2
  Sin : Inport  Port=3
  Enable : EnablePort
  Complex to Real-Imag : ComplexToRealImag
  Demux : Demux
  Mux : Mux  Inputs=2
  Mux1 : Mux  Inputs=3
  Real-Imag to Complex : RealImagToComplex
  Real-Imag to Complex1 : RealImagToComplex
  S-Function : S-Function  FunctionName=s_power_flow_fault_gs_nr  Parameters=genTranReactance,faultaugYMatrix,no_gen_co,no_gen_wi,noGridNodes,2  EnableBusSupport=off
  Vout : Outport
  Sout : Outport  Port=2
  wires:
  E/1 -> Mux1/1
  Sin/1 -> Mux1/3
  V/1 -> Mux1/2
  S-Function/1 -> Demux/1
  Mux1/1 -> Complex to Real-Imag/1
  Mux/1 -> S-Function/1
  Complex to Real-Imag/1 -> Mux/1
  Complex to Real-Imag/2 -> Mux/2
  Demux/1 -> Real-Imag to Complex/1
  Demux/2 -> Real-Imag to Complex/2
  Real-Imag to Complex/1 -> Vout/1
  Demux/3 -> Real-Imag to Complex1/1
  Demux/4 -> Real-Imag to Complex1/2
  Real-Imag to Complex1/1 -> Sout/1

== system wtd_library_ver1/WTD Network ver1/power_flow_fault1 ==
  E : Inport
  V : Inport  Port=2
  Sin : Inport  Port=3
  Enable : EnablePort
  Complex to Real-Imag : ComplexToRealImag
  Demux : Demux
  Mux : Mux  Inputs=2
  Mux1 : Mux  Inputs=3
  Real-Imag to Complex : RealImagToComplex
  Real-Imag to Complex1 : RealImagToComplex
  S-Function1 : S-Function  FunctionName=s_power_flow_fault_gs_nr  Parameters=genTranReactance,clearaugYMatrix,no_gen_co,no_gen_wi,noGridNodes,2  EnableBusSupport=off
  Vout : Outport
  Sout : Outport  Port=2
  wires:
  Real-Imag to Complex1/1 -> Sout/1
  Demux/4 -> Real-Imag to Complex1/2
  Demux/3 -> Real-Imag to Complex1/1
  Real-Imag to Complex/1 -> Vout/1
  Demux/2 -> Real-Imag to Complex/2
  Demux/1 -> Real-Imag to Complex/1
  Complex to Real-Imag/2 -> Mux/2
  Complex to Real-Imag/1 -> Mux/1
  Mux/1 -> S-Function1/1
  Mux1/1 -> Complex to Real-Imag/1
  S-Function1/1 -> Demux/1
  V/1 -> Mux1/2
  Sin/1 -> Mux1/3
  E/1 -> Mux1/1

== system wtd_library_ver1/WTD PLL ver1/alpa_beta to dq ==
  angle(V) : Inport
  Gain1 : Gain
  Gain2 : Gain  Gain=-1
  Matrix Concatenate : Concatenate  Mode=Multidimensional array
  Reshape : Reshape  OutputDimensionality=Customize  OutputDimensions=[1,2]
  Reshape1 : Reshape  OutputDimensionality=Customize  OutputDimensions=[1,2]
  Trigonometric Function : Trigonometry  Operator=cos
  Trigonometric Function1 : Trigonometry
  Trigonometric Function2 : Trigonometry
  Trigonometric Function3 : Trigonometry  Operator=cos
  Vector Concatenate : Concatenate
  Vector Concatenate1 : Concatenate
  matT : Outport
  wires:
  angle(V)/1 -> Trigonometric Function/1, Trigonometric Function1/1, Trigonometric Function3/1, Trigonometric Function2/1
  Trigonometric Function/1 -> Vector Concatenate/1
  Trigonometric Function1/1 -> Vector Concatenate/2
  Trigonometric Function2/1 -> Gain2/1
  Trigonometric Function3/1 -> Gain1/1
  Gain1/1 -> Vector Concatenate1/2
  Vector Concatenate/1 -> Reshape/1
  Vector Concatenate1/1 -> Reshape1/1
  Reshape/1 -> Matrix Concatenate/1
  Reshape1/1 -> Matrix Concatenate/2
  Matrix Concatenate/1 -> matT/1
  Gain2/1 -> Vector Concatenate1/1

== system wtd_library_ver1/WTD Thermo ver1/Rotor//Load1 ==
  note: This subsystem models the mechanical part of the synchronous machine (Kundur)
  "deltaPe(pu) " : Inport  PortDimensions=1
  deltaPm(pu) : Inport  Port=2  PortDimensions=1
  angle(E)(elrad) : Inport  Port=3  PortDimensions=1
  deltawro : Inport  Port=4  PortDimensions=1
  Constant : Constant
  F1 : Gain  Gain=D2  SaturateOnIntegerOverflow=on  OutDataTypeStr=Inherit: Same as input  ParamDataTypeStr=Inherit: Same as input
  H : Constant  Value=H2
  Integrator : Integrator  InitialConditionSource=external  InitialCondition=dwo
  Integrator2 : Integrator  InitialConditionSource=external  InitialCondition=tho
  Product1 : Product  Inputs=*/  SaturateOnIntegerOverflow=on  InputSameDT=on  OutDataTypeStr=Inherit: Same as first input
  Product2 : Product  Inputs=*/  SaturateOnIntegerOverflow=on  InputSameDT=on  OutDataTypeStr=Inherit: Same as first input
  Sum1 : Sum  Inputs=+-  SaturateOnIntegerOverflow=on  InputSameDT=on  OutDataTypeStr=Inherit: Same as first input
  Sum2 : Sum  Inputs=+-  SaturateOnIntegerOverflow=on  InputSameDT=on  OutDataTypeStr=Inherit: Same as first input
  Sum3 : Sum  SaturateOnIntegerOverflow=on  InputSameDT=on  OutDataTypeStr=Inherit: Same as first input
  gain : Gain  Gain=2  SaturateOnIntegerOverflow=on  OutDataTypeStr=Inherit: Same as input  ParamDataTypeStr=Inherit: Same as input
  wbase : Gain  Gain=wbase  SaturateOnIntegerOverflow=on  OutDataTypeStr=Inherit: Same as input  ParamDataTypeStr=Inherit: Same as input
  delta(elrad) : Outport  InitialOutput=0
  delta_w(pu) : Outport  Port=2  InitialOutput=0
  wires:
  deltaPm(pu)/1 -> Sum2/1
  Sum3/1 -> Product2/2
  Constant/1 -> Sum3/1
  Product2/1 -> Sum1/1
  Sum2/1 -> Product2/1
  F1/1 -> Sum1/2
  Sum1/1 -> Product1/1
  gain/1 -> Product1/2
  deltawro/1 -> Integrator/2
  angle(E)(elrad)/1 -> Integrator2/2
  Integrator2/1 -> delta(elrad)/1  "delta (rad)"
  wbase/1 -> Integrator2/1  "delta_w"
  Integrator/1 -> Sum3/2, delta_w(pu)/1, F1/1, wbase/1  "dw"
  Product1/1 -> Integrator/1
  "deltaPe(pu) "/1 -> Sum2/2  "Pe"
  H/1 -> gain/1

== system wtd_library_ver1/WTD Thermo ver1/TGOV1 ==
  note: MODEL PSS: TGOV1
  Pinit (pu mach) : Inport
  deltaw : Inport  Port=2
  Add : Sum  Inputs=+-
  Add1 : Sum  Inputs=+-
  Add2 : Sum  Inputs=++-
  Add3 : Sum  Inputs=+-
  Gain : Gain  Gain=1/R2
  Gain1 : Gain  Gain=1/T12
  Gain2 : Gain  Gain=1/T32
  Gain3 : Gain  Gain=T22
  Gain4 : Gain  Gain=Dt2
  Gain5 : Gain  Gain=R2
  Integrator : Integrator  InitialConditionSource=external  LimitOutput=on  UpperSaturationLimit=Vmax2  LowerSaturationLimit=Vmin2
  Integrator1 : Integrator  InitialConditionSource=external
  PMECH : Outport
  wires:
  Gain/1 -> Add/1
  Add/1 -> Gain1/1
  Gain1/1 -> Integrator/1
  Pinit (pu mach)/1 -> Integrator1/2, Integrator/2, Gain5/1
  Integrator/1 -> Add/2, Add1/1
  Add1/1 -> Gain2/1
  Gain2/1 -> Integrator1/1, Gain3/1
  Integrator1/1 -> Add1/2, Add2/2
  Gain3/1 -> Add2/1
  Add2/1 -> PMECH/1
  Gain4/1 -> Add2/3
  deltaw/1 -> Gain4/1, Add3/2
  Add3/1 -> Gain/1
  Gain5/1 -> Add3/1

== system wtd_library_ver1/WTD Wind Turbine ver1_1/cp(lambda,beta)1 ==
  lambda : Inport
  beta : Inport  Port=2
  Fcn : Fcn  Expr=1/(1/(u[1]+0.08*u[2])-0.035/(u[2]^3+1))
  Fcn1 : Fcn  Expr=c1*(c2/u[2]-c3*u[3]-c4)*exp(-c5/u[2])+c6*u[1]
  Mux : Mux  Inputs=2
  Mux1 : Mux  Inputs=3
  cp : Outport
  wires:
  Mux/1 -> Fcn/1
  beta/1 -> Mux/2, Mux1/3
  Mux1/1 -> Fcn1/1
  lambda/1 -> Mux/1, Mux1/1
  Fcn1/1 -> cp/1
  Fcn/1 -> Mux1/2  "lambda_i"

== system wtd_library_ver1/WTD DFIG_ver1/Converter control model/Electrical Control ==
  Qcmd : Inport
  Qgen : Inport  Port=2
  Vterm : Inport  Port=3
  Pord : Inport  Port=4
  Aux_Test_Sig : Inport  Port=5
  Add : Sum  Inputs=-+
  Add1 : Sum
  Add5 : Sum  Inputs=++-
  Divide : Product  Inputs=*/
  Gain : Gain  Gain=KQi
  Gain1 : Gain  Gain=KVi
  Gain2 : Gain  Gain=KPiadd
  IPmax limit : Saturate  UpperLimit=IPmax  LowerLimit=-inf
  s0cc : Integrator  InitialCondition=s0cc  LimitOutput=on  UpperSaturationLimit=Vmax  LowerSaturationLimit=Vmin
  s1cc : Integrator  InitialCondition=s1cc  LimitOutput=on  UpperSaturationLimit=XIQmax  LowerSaturationLimit=XIQmin
  Eqcmd : Outport
  Ipcmd : Outport  Port=2
  wires:
  Add1/1 -> Eqcmd/1
  Gain2/1 -> Add1/1
  s1cc/1 -> Add1/2
  IPmax limit/1 -> Ipcmd/1
  Divide/1 -> IPmax limit/1
  Pord/1 -> Divide/1
  Vterm/1 -> Add5/3, Divide/2
  Aux_Test_Sig/1 -> Add5/1
  Gain1/1 -> s1cc/1
  Add5/1 -> Gain2/1, Gain1/1
  s0cc/1 -> Add5/2  "Vref"
  Gain/1 -> s0cc/1
  Qgen/1 -> Add/1
  Qcmd/1 -> Add/2
  Add/1 -> Gain/1

== system wtd_library_ver1/WTD DFIG_ver1/Converter control model/Reactive Power Control ==
  Vrfq : Inport
  Vreg : Inport  Port=2
  Qord_sep_mod : Inport  Port=3
  PFAref : Inport  Port=4
  Pelec : Inport  Port=5
  Qinput_droop : Inport  Port=6
  Qref : Inport  Port=7
  Power Factor Regulator : Subsystem
  Wind Control Emulator : Subsystem
  Qcmd : Outport
  wires:
  Qref/1 -> Power Factor Regulator/4(Qref)
  Pelec/1 -> Power Factor Regulator/2(Pelec)
  Qord_sep_mod/1 -> Power Factor Regulator/5(Qord_sep_mod)
  PFAref/1 -> Power Factor Regulator/1(PFAref)
  Wind Control Emulator/1(Qord) -> Power Factor Regulator/3(Qord)
  Power Factor Regulator/1(Qcmd) -> Qcmd/1
  Qinput_droop/1 -> Wind Control Emulator/3(Qinput)
  Vreg/1 -> Wind Control Emulator/2(Vreg)
  Vrfq/1 -> Wind Control Emulator/1(Vrfq)

== system wtd_library_ver1/WTD DFIG_ver1/Generator_converter_model/ Transformation1 ==
  note: Isorc = ((P+jQ)/V)*
  -Iq*Vt = Qelec : Inport
  Ip*Vt : Inport  Port=2
  V : Inport  Port=3
  Add : Sum
  Constant : Constant  Value=j
  Divide1 : Product  Inputs=*/
  Divide3 : Product  Inputs=**
  Math Function1 : Math  Operator=conj  SaturateOnIntegerOverflow=on
  Isorc : Outport
  wires:
  V/1 -> Divide1/2
  Constant/1 -> Divide3/1
  Ip*Vt/1 -> Add/2  "Pelec"
  -Iq*Vt = Qelec/1 -> Divide3/2
  Divide1/1 -> Math Function1/1
  Divide3/1 -> Add/1  "Qelec"
  Add/1 -> Divide1/1
  Math Function1/1 -> Isorc/1

== system wtd_library_ver1/WTD DFIG_ver1/Generator_converter_model/High voltage reactive current management ==
  note: signs reversed
      |  (in comparison to Ref. 71)
  note: -IqVt
  Eq : Inport
  absV : Inport  Port=2
  absXsec : Inport  Port=3
  Add1 : Sum  Inputs=+-
  Add2 : Sum  Inputs=+-
  Constant1 : Constant  Value=volim
  Constant2 : Constant  Value=0
  Divide2 : Product  Inputs=/*
  Divide3 : Product  Inputs=**
  Gain2 : Gain  Gain=khv
  Gain3 : Gain  Gain=+1
  Saturation1 : Saturate  UpperLimit=inf  LowerLimit=0
  Saturation2 : Saturate  UpperLimit=iolim  LowerLimit=-inf
  Switch : Switch  Criteria=u2 > Threshold
  Terminator : Terminator
  -Iq*Vt_limit : Outport
  wires:
  absV/1 -> Divide3/2, Add1/1
  Constant1/1 -> Add1/2
  Add1/1 -> Gain2/1, Switch/2
  Eq/1 -> Divide2/2
  Divide2/1 -> Gain3/1
  absXsec/1 -> Divide2/1
  Add2/1 -> -Iq*Vt_limit/1
  Gain2/1 -> Saturation1/1
  Divide3/1 -> Add2/1
  Saturation1/1 -> Switch/1
  Constant2/1 -> Switch/3
  Switch/1 -> Add2/2
  Gain3/1 -> Divide3/1, Saturation2/1
  Saturation2/1 -> Terminator/1

== system wtd_library_ver1/WTD DFIG_ver1/Generator_converter_model/Low voltage active current management ==
  Ip : Inport
  absV : Inport  Port=2
  Add : Sum
  Constant1 : Constant  Value=nlvacm
  Constant2 : Constant  Value=0
  Divide1 : Product  Inputs=**
  Divide3 : Product  Inputs=**
  Gain1 : Gain  Gain=klvacm
  Saturation : Saturate  UpperLimit=1  LowerLimit=0
  Switch : Switch  Threshold=lvpnt1
  Switch2 : Switch  Criteria=u2 > Threshold  Threshold=lvpnt0
  Ip*Vt_limit : Outport
  wires:
  Constant1/1 -> Add/2
  Add/1 -> Saturation/1
  Gain1/1 -> Add/1
  Ip/1 -> Divide3/1
  absV/1 -> Gain1/1, Switch/2, Switch/1, Switch2/2, Divide1/1
  Switch2/1 -> Switch/3
  Saturation/1 -> Divide1/2
  Constant2/1 -> Switch2/3
  Divide3/1 -> Ip*Vt_limit/1
  Divide1/1 -> Switch2/1
  Switch/1 -> Divide3/2

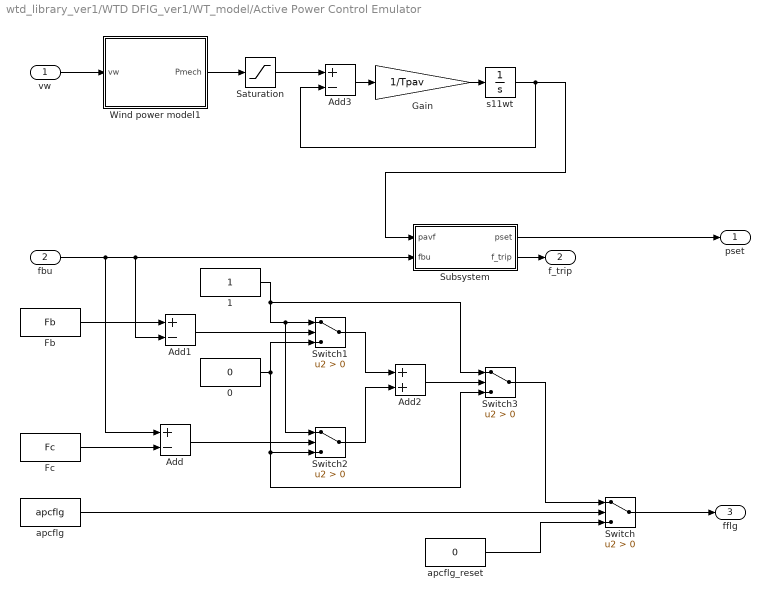
== system wtd_library_ver1/WTD DFIG_ver1/WT_model/Active Power Control Emulator ==
  vw : Inport
  fbu : Inport  Port=2
  0 : Constant  Value=0
  1 : Constant
  Add : Sum  Inputs=+-
  Add1 : Sum  Inputs=+-
  Add2 : Sum
  Add3 : Sum  Inputs=+-
  Fb : Constant  Value=Fb
  Fc : Constant  Value=Fc
  Gain : Gain  Gain=1/Tpav
  Saturation : Saturate  UpperLimit=Prated  LowerLimit=-inf
  Subsystem : Subsystem
  Switch{,1..3} (4 alike) : Switch  Criteria=u2 > Threshold
  Wind power model1 : Subsystem
  apcflg : Constant  Value=apcflg
  apcflg_reset : Constant  Value=0
  s11wt : Integrator  InitialCondition=s11wt
  pset : Outport
  f_trip : Outport  Port=2
  fflg : Outport  Port=3
  wires:
  Saturation/1 -> Add3/1
  s11wt/1 -> Subsystem/1(pavf), Add3/2
  Gain/1 -> s11wt/1
  Add3/1 -> Gain/1
  Switch3/1 -> Switch/1
  Add2/1 -> Switch3/2
  Switch2/1 -> Add2/2
  Switch1/1 -> Add2/1
  Add/1 -> Switch2/2
  0/1 -> Switch3/3, Switch2/3, Switch1/3
  1/1 -> Switch3/1, Switch2/1, Switch1/1
  Add1/1 -> Switch1/2
  Fb/1 -> Add1/1
  Fc/1 -> Add/2
  Subsystem/1(pset) -> pset/1
  Switch/1 -> fflg/1
  apcflg_reset/1 -> Switch/3
  apcflg/1 -> Switch/2
  Subsystem/2(f_trip) -> f_trip/1
  fbu/1 -> Add1/2, Subsystem/2(fbu), Add/1
  Wind power model1/1(Pmech) -> Saturation/1
  vw/1 -> Wind power model1/1(vw)

== system wtd_library_ver1/WTD DFIG_ver1/WT_model/Pitch compensator ==
  Perr : Inport
  theta2_0 : Inport  Port=2
  Antiwindupin : Inport  Port=3
  Add : Sum
  Constant : Constant  Value=thetamin
  Constant1 : Constant  Value=thetamax
  Divide : Product  Inputs=**  OutDataTypeStr=double
  Gain : Gain  Gain=Kic
  Gain1 : Gain  Gain=Kpc
  Integrator : Integrator  InitialConditionSource=external
  Saturation : Subsystem
  theta2 : Outport
  wires:
  Antiwindupin/1 -> Saturation/4(y)
  Saturation/1(ysw) -> Divide/2
  Constant1/1 -> Saturation/2(ymax)
  Constant/1 -> Saturation/3(ymin)
  theta2_0/1 -> Integrator/2
  Divide/1 -> Integrator/1
  Gain/1 -> Divide/1
  Add/1 -> theta2/1
  Gain1/1 -> Add/1
  Perr/1 -> Saturation/1(z), Gain/1, Gain1/1
  Integrator/1 -> Add/2

== system wtd_library_ver1/WTD DFIG_ver1/WT_model/Pitch controller ==
  werr : Inport
  theta1_0 : Inport  Port=2
  Antiwindupin : Inport  Port=3
  Add : Sum
  Constant : Constant  Value=thetamin
  Constant1 : Constant  Value=thetamax
  Divide : Product  Inputs=**  OutDataTypeStr=double
  Gain : Gain  Gain=Kip
  Gain1 : Gain  Gain=Kpp
  Integrator : Integrator  InitialConditionSource=external
  Saturation : Subsystem
  theta1 : Outport
  wires:
  Saturation/1(ysw) -> Divide/2
  Antiwindupin/1 -> Saturation/4(y)
  Constant1/1 -> Saturation/2(ymax)
  Constant/1 -> Saturation/3(ymin)
  Divide/1 -> Integrator/1
  Gain/1 -> Divide/1
  theta1_0/1 -> Integrator/2
  Integrator/1 -> Add/2
  werr/1 -> Saturation/1(z), Gain/1, Gain1/1
  Gain1/1 -> Add/1
  Add/1 -> theta1/1

== system wtd_library_ver1/WTD DFIG_ver1/WT_model/Pitch model ==
  thetacmd : Inport
  theta0 : Inport  Port=2
  Add : Sum  Inputs=+-
  Gain : Gain  Gain=1/Tp
  Integrator : Integrator  InitialConditionSource=external  LimitOutput=on  UpperSaturationLimit=thetamax  LowerSaturationLimit=thetamin
  dtheta/dtmax_min : Saturate  UpperLimit=dtheta_dtmax  LowerLimit=dtheta_dtmin
  theta : Outport
  wires:
  dtheta/dtmax_min/1 -> Integrator/1
  thetacmd/1 -> Add/1
  Add/1 -> Gain/1
  Gain/1 -> dtheta/dtmax_min/1
  theta0/1 -> Integrator/2
  Integrator/1 -> theta/1, Add/2

== system wtd_library_ver1/WTD DFIG_ver1/WT_model/Plim ==
  Pcmd : Inport
  Pord0 : Inport  Port=2
  Add : Sum  Inputs=+-
  Gain : Gain  Gain=1/Tpc
  Integrator : Integrator  InitialConditionSource=external  LimitOutput=on  UpperSaturationLimit=Pwmax  LowerSaturationLimit=Pwmin
  dP/dtmax_min : Saturate  UpperLimit=dP_dtmax  LowerLimit=dP_dtmin
  Pinp : Outport
  wires:
  Gain/1 -> dP/dtmax_min/1
  dP/dtmax_min/1 -> Integrator/1
  Integrator/1 -> Add/2, Pinp/1
  Pord0/1 -> Integrator/2
  Add/1 -> Gain/1
  Pcmd/1 -> Add/1

== system wtd_library_ver1/WTD DFIG_ver1/WT_model/Plim1 ==
  word : Inport
  wordf0 : Inport  Port=2
  Add : Sum  Inputs=+-
  Gain : Gain  Gain=1/60
  Integrator : Integrator  InitialConditionSource=external
  wordf : Outport
  wires:
  word/1 -> Add/1
  Add/1 -> Gain/1
  Gain/1 -> Integrator/1
  wordf0/1 -> Integrator/2
  Integrator/1 -> wordf/1, Add/2

== system wtd_library_ver1/WTD DFIG_ver1/WT_model/Power_Response_Rate_Limiter ==
  pinp : Inport
  pstl : Inport  Port=2
  dpwi : Inport  Port=3
  Add : Sum  Inputs=+-
  Add1 : Sum  Inputs=-+
  Add2 : Sum  Inputs=+-
  Add3 : Sum  Inputs=+++
  Gain : Gain  Gain=1/Tw
  Switch : Switch  Criteria=u2 > Threshold
  s10wt : Integrator  InitialCondition=s10wt
  Pord : Outport
  wires:
  dpwi/1 -> Add3/3
  Add3/1 -> Pord/1
  s10wt/1 -> Gain/1
  Add2/1 -> Add3/1, s10wt/1  "wsho"
  Add/1 -> Add2/1  "perr"
  Gain/1 -> Add2/2
  Switch/1 -> Add3/2, Add/2  "plim"
  Add1/1 -> Switch/2
  pstl/1 -> Switch/3, Add1/2
  pinp/1 -> Add/1, Switch/1, Add1/1

== system wtd_library_ver1/WTD DFIG_ver1/WT_model/Rotor model ==
  note: deltaw(pu)
  Pa : Inport
  deltaw0(pu) : Inport  Port=2
  Add : Sum
  Divide : Product  Inputs=*/
  Gain : Gain  Gain=1/(2*H)
  Integrator : Integrator  InitialConditionSource=external
  s6wt : Constant  Value=s6wt
  w : Outport
  wires:
  s6wt/1 -> Add/2
  Add/1 -> Divide/2, w/1
  deltaw0(pu)/1 -> Integrator/2
  Pa/1 -> Divide/1
  Integrator/1 -> Add/1
  Gain/1 -> Integrator/1
  Divide/1 -> Gain/1

== system wtd_library_ver1/WTD DFIG_ver1/WT_model/Torque controller ==
  werr : Inport
  Tcmd0 : Inport  Port=2
  Antiwindupin : Inport  Port=3
  Add : Sum
  Constant : Constant  Value=Pwmax
  Constant1 : Constant  Value=Pwmin
  Divide : Product  Inputs=**  OutDataTypeStr=double
  Gain : Gain  Gain=Kitrq
  Gain1 : Gain  Gain=Kptrq
  Integrator : Integrator  InitialConditionSource=external
  Saturation : Subsystem
  Tcmd : Outport
  wires:
  Antiwindupin/1 -> Saturation/4(y)
  Saturation/1(ysw) -> Divide/2
  Constant1/1 -> Saturation/3(ymin)
  Constant/1 -> Saturation/2(ymax)
  Gain/1 -> Divide/1
  Divide/1 -> Integrator/1
  Add/1 -> Tcmd/1
  Gain1/1 -> Add/1
  werr/1 -> Saturation/1(z), Gain/1, Gain1/1
  Integrator/1 -> Add/2
  Tcmd0/1 -> Integrator/2

== system wtd_library_ver1/WTD DFIG_ver1/WT_model/Under Speed Trip ==
  w : Inport
  Add : Sum  Inputs=+-
  Constant1 : Constant
  Constant2 : Constant  Value=0
  Switch : Switch
  wlow : Constant  Value=0.1
  w_trip : Outport
  wires:
  Switch/1 -> w_trip/1
  Constant2/1 -> Switch/3
  Constant1/1 -> Switch/1
  Add/1 -> Switch/2
  w/1 -> Add/2
  wlow/1 -> Add/1

== system wtd_library_ver1/WTD DFIG_ver1/WT_model/Wind power model ==
  theta : Inport
  vw : Inport  Port=2
  w : Inport  Port=3
  Cp & lambda : Subsystem
  Divide1 : Product  Inputs=***
  Fcn : Fcn  Expr=u^3
  Ka : Constant  Value=Ka(co_node)
  Reshape : Reshape
  Pmech : Outport
  Cp : Outport  Port=2
  lambda : Outport  Port=3
  wires:
  Reshape/1 -> Cp/1, Divide1/2
  Cp & lambda/2(lambda) -> lambda/1
  Divide1/1 -> Pmech/1  "Pmech"
  w/1 -> Cp & lambda/3(w)
  theta/1 -> Cp & lambda/1(theta)
  Fcn/1 -> Divide1/1
  Cp & lambda/1(Cp) -> Reshape/1
  Ka/1 -> Divide1/3
  vw/1 -> Fcn/1, Cp & lambda/2(vw)

== system wtd_library_ver1/WTD DFIG_ver1/WT_model/WindInertia Control ==
  note: dbwi
  fbus : Inport
  fref : Inport  Port=2
  Add : Sum  Inputs=-+
  Add1 : Sum  Inputs=+-
  Add2 : Sum  Inputs=+-
  Dead Zone : DeadZone  LowerValue=0  UpperValue=dbwi  SaturateOnIntegerOverflow=on
  Gain : Gain  Gain=1/TIpwi
  Gain1 : Gain  Gain=Kwi
  Gain2 : Gain  Gain=1/Twowi
  Rate Limiter1 : RateLimiter  RisingSlewLimit=urlwi  FallingSlewLimit=drlwi  SampleTimeMode=inherited
  Saturation2 : Saturate  UpperLimit=Pmxwi  LowerLimit=Pmnwi
  s12wt : Integrator  InitialCondition=s12wt
  s13wt : Integrator  InitialCondition=s13wt
  dpwi : Outport
  wires:
  Add2/1 -> s13wt/1, Rate Limiter1/1
  Rate Limiter1/1 -> Saturation2/1
  Saturation2/1 -> dpwi/1
  s13wt/1 -> Gain2/1
  Gain2/1 -> Add2/2
  Gain1/1 -> Add2/1
  s12wt/1 -> Add1/2, Gain1/1
  Dead Zone/1 -> Add1/1
  Add1/1 -> Gain/1
  Gain/1 -> s12wt/1
  Add/1 -> Dead Zone/1  "ferrwi"
  fref/1 -> Add/2
  fbus/1 -> Add/1

== system wtd_library_ver1/WTD Hydro ver1/HYDRO turbine _HYGOV/Integrator and limits ==
  Filter in : Inport
  Kplus11 : Inport  Port=2
  Gain2 : Gain  Gain=1/(r1*Tr1)
  Saturation : Saturate  UpperLimit=VELM1  LowerLimit=-VELM1
  gate_ref : Integrator  InitialConditionSource=external  LimitOutput=on  UpperSaturationLimit=Gmax1  LowerSaturationLimit=Gmin1
  Valve out : Outport
  wires:
  Filter in/1 -> Gain2/1
  Gain2/1 -> Saturation/1
  gate_ref/1 -> Valve out/1
  Saturation/1 -> gate_ref/1
  Kplus11/1 -> gate_ref/2
